simulink model "lab4_3"  (R2021b)
settings: Solver=VariableStepAuto  StartTime=0.0  StopTime=10.0  RelTol=1e-3
values from neighbouring files (symbols this model uses):
  K = rlocfind(G)    [s2_1.m]    (also in s2_2.m; s2_3.m)
  Ti = TI    (= 0.0835625)    [s2_2.m]    (also in s2_3.m = 0.059361)
  VMAX_UPM = 11.75    [s2_2.m]    (also in s2_3.m)
libraries: nonlinear_cart_lab4 x1
settings Model: Creator=adanm  LastModifiedBy=Juho
settings SolverCC: AlgebraicLoopSolver=TrustRegion
settings DataIOCC: ReturnWorkspaceOutputs=off
settings DebuggingCC: SFMachineParentedDataDiag=warning  ArithmeticOperatorsInVariantConditions=warning
settings SFSimCC: CustomCodeUndefinedFunction=UseInterfaceOnly

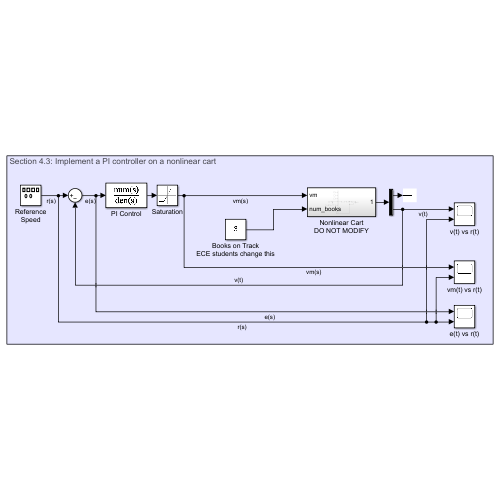
[thumbnail: Simulink's stored preview of the top-level diagram]
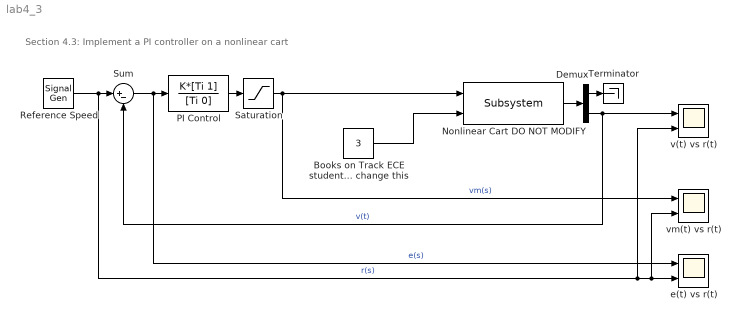
== system lab4_3 ==
  note: Section 4.3: Implement a PI controller on a nonlinear cart
  Books on Track ECE students change this : Constant  Value=3  OutMin=[0]  OutMax=[10]
  Demux : Demux  Outputs=2
  Nonlinear Cart DO NOT MODIFY : nonlinear_cart_lab4/Subsystem  SystemSampleTime=-1  VariantActivationTime=update diagram  Latency=0  AutoFrameSizeCalculation=off
  PI Control : TransferFcn  Numerator=K*[Ti 1]  Denominator=[Ti 0]
  Reference Speed : SignalGenerator  WaveForm=square  Amplitude=0.2  Frequency=0.5
  "Saturation " : Saturate  UpperLimit=VMAX_UPM  LowerLimit=-VMAX_UPM
  Sum : Sum  Inputs=|+-
  Terminator : Terminator
  e(t) vs r(t) : Scope  NumInputPorts=2
  v(t) vs r(t) : Scope  NumInputPorts=2
  vm(t) vs r(t) : Scope  NumInputPorts=2
  wires:
  Reference Speed/1 -> v(t) vs r(t)/2, vm(t) vs r(t)/2, e(t) vs r(t)/2, Sum/1  "r(s)"
  Sum/1 -> e(t) vs r(t)/1, PI Control/1  "e(s)"
  PI Control/1 -> "Saturation "/1
  "Saturation "/1 -> Nonlinear Cart DO NOT MODIFY/1, vm(t) vs r(t)/1  "vm(s)"
  Nonlinear Cart DO NOT MODIFY/1 -> Demux/1
  Demux/2 -> v(t) vs r(t)/1, Sum/2  "v(t)"
  Demux/1 -> Terminator/1
  Books on Track ECE students change this/1 -> Nonlinear Cart DO NOT MODIFY/2
